simulink model "Grid_Connected_VSM"  (R2018a)
settings: Solver=ode45  StartTime=0.0  StopTime=0.6  RelTol=1e-3
InitFcn:
  | clear all;
  | Vdc = 1200;
  | fc = 10e3;
  | Rf = 0.07;
  | Lf = 5.2e-3;
  | Cf = 100e-6;
  | Lc = 1.5e-4;
  | Rc = 0.05;
  | Vref = sqrt(2/3)*400;
  | 
  | Kpv = 3;
  | Kiv = 400;
  | Kpc = 5;
  | Kic = 10;
  | 
  | 
  | J=0.05;
  | D=10;
  | %D = 1000;
  | wn=2*pi*50;
  | wf = 10*pi;
  | mq = 1e-5;
undefined symbols (not defined in the file): R2
libraries: powerlib x13, powerlib_meascontrol x5, simulink x4
settings Model: SimulationMode=accelerator  Creator=Deependra  LastModifiedBy=Deependra

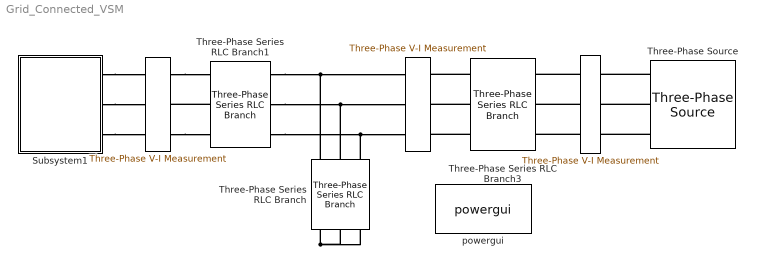
== system Grid_Connected_VSM ==
  " " : powerlib/Measurements/Three-Phase V-I Measurement  VoltageMeasurement=phase-to-ground  SetLabelV=on  LabelV=Viabc  Vpu=off  VpuLL=off  CurrentMeasurement=yes  SetLabelI=on  LabelI=ILabc  Ipu=off  Pbase=100e6  Vbase=500e3  OutputType=Complex  PhasorSimulation=off  PSBequivalent=0
  "   " : powerlib/Measurements/Three-Phase V-I Measurement  VoltageMeasurement=phase-to-ground  SetLabelV=on  LabelV=Voabc  Vpu=off  VpuLL=off  CurrentMeasurement=yes  SetLabelI=on  LabelI=Ioabc  Ipu=off  Pbase=Pnom  Vbase=380  OutputType=Complex  PhasorSimulation=off  PSBequivalent=0
  "     " : powerlib/Measurements/Three-Phase V-I Measurement  VoltageMeasurement=phase-to-ground  SetLabelV=on  LabelV=Vg  Vpu=off  VpuLL=off  CurrentMeasurement=no  SetLabelI=off  LabelI=Iabc_0  Ipu=off  Pbase=Pnom  Vbase=380  OutputType=Complex  PhasorSimulation=off  PSBequivalent=0
  Subsystem1 : Subsystem
  Three-Phase Series RLC Branch : powerlib/Elements/Three-Phase Series RLC Branch  LConnTagsString=A|B|C  RConnTagsString=A|B|C  BranchType=C  Resistance=R2  Inductance=1e-3  Capacitance=Cf  Measurements=Branch voltages
  Three-Phase Series RLC Branch1 : powerlib/Elements/Three-Phase Series RLC Branch  LConnTagsString=A|B|C  RConnTagsString=A|B|C  BranchType=RL  Resistance=Rf  Inductance=Lf  Capacitance=4.5e-3  Measurements=Branch voltages
  Three-Phase Series RLC Branch3 : powerlib/Elements/Three-Phase Series RLC Branch  LConnTagsString=A|B|C  RConnTagsString=A|B|C  BranchType=RL  Resistance=Rc  Inductance=Lc  Capacitance=1e-6  Measurements=None
  Three-Phase Source : powerlib/Electrical Sources/Three-Phase Source  InternalConnection=Yg  VoltagePhases=off  Voltage=400  PhaseAngle=0  Voltage_phases=[25e3 25e3 25e3]/sqrt(3)  PhaseAngles_phases=[0 -120 +120]  Frequency=50  NonIdealSource=off  SpecifyImpedance=off  Resistance=0.8929  Inductance=16.58e-3  ShortCircuitLevel=100e6  BaseVoltage=25e3  XRratio=7  BusType=swing  Pref=10e3  Qref=0  Prefabc=[10e3, 10e3, 10e3]  Qrefabc=[0, 0, 0]  Qmin=-inf  Qmax=inf
  powergui : powerlib/powergui  Priority=1  SimulationMode=Discrete  SampleTime=5e-6  frequency=60  Iterations=50  frequencyindice=0  Pbase=100e6  ErrMax=1e-4  UnitsV=kV  UnitsW=MW  buscounter=0  FunctionMessages=off  echomessages=off  EnableUseOfTLC=off  CurrentSourceSwitches=off  DisableSnubberDevices=off  DisableRonSwitches=off  DisableVfSwitches=off  DisplayEquations=off  SolverType=Tustin/Backward Euler (TBE)  Interpol=off  ExternalGateDelay=off  methode=off  Ts=100  x0status=zero  SPID=off  SwTol=0  HookPort=off  RestoreLinks=warning  ResistiveCurrentMeasurement=off  Frange=[0:2:500]  Ylog=off  Xlog=on  ShowGrid=off  save=off  variable=ZData  structure=Ni  ZoomFFT=off  StartTime=0.6  cycles=10  DisplayStyle=1  fundamental=50  FreqAxis=off  MaxFrequency=1000  frequencyindicesteady=1  RmsSteady=1  display=off
  connections:
  Three-Phase Series RLC Branch/LConn1 -- Three-Phase Series RLC Branch1/RConn1 -- "   "/LConn1
  Three-Phase Series RLC Branch/LConn3 -- Three-Phase Series RLC Branch1/RConn3 -- "   "/LConn3
  Three-Phase Series RLC Branch/RConn1 -- Three-Phase Series RLC Branch/RConn2 -- Three-Phase Series RLC Branch/RConn3
  Three-Phase Series RLC Branch/LConn2 -- Three-Phase Series RLC Branch1/RConn2 -- "   "/LConn2
  Three-Phase Series RLC Branch3/LConn3 -- "   "/RConn3
  Three-Phase Series RLC Branch3/LConn1 -- "   "/RConn1
  "     "/LConn2 -- Three-Phase Series RLC Branch3/RConn2
  "     "/LConn1 -- Three-Phase Series RLC Branch3/RConn1
  Three-Phase Series RLC Branch3/LConn2 -- "   "/RConn2
  "     "/LConn3 -- Three-Phase Series RLC Branch3/RConn3
  Subsystem1/RConn1 -- " "/LConn1
  Subsystem1/RConn2 -- " "/LConn2
  Subsystem1/RConn3 -- " "/LConn3
  Three-Phase Source/RConn2 -- "     "/RConn2
  Three-Phase Source/RConn1 -- "     "/RConn1
  Three-Phase Source/RConn3 -- "     "/RConn3
  " "/RConn1 -- Three-Phase Series RLC Branch1/LConn1
  Three-Phase Series RLC Branch1/LConn2 -- " "/RConn2
  " "/RConn3 -- Three-Phase Series RLC Branch1/LConn3

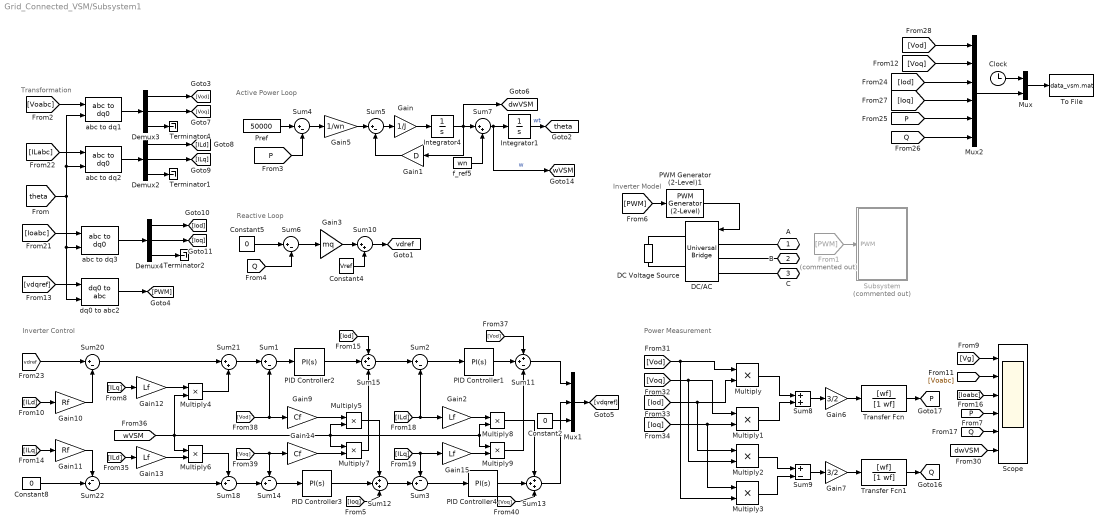
== system Grid_Connected_VSM/Subsystem1 ==
  note: Power Measurement
  note: Inverter Control
  note: Reactive Loop
  note: Transformation
  note: Active Power Loop
  note: Inverter Model
  Clock : Clock
  Constant2 : Constant  Value=0
  Constant4 : Constant  Value=Vref
  Constant5 : Constant  Value=0
  Constant8 : Constant  Value=0
  DC Voltage Source : powerlib/Electrical Sources/DC Voltage Source  Amplitude=Vdc  Measurements=None
  DC/AC : powerlib/Power Electronics/Universal Bridge  Arms=3  SnubberResistance=1e5  SnubberCapacitance=inf  Device=IGBT / Diodes  Ron=1e-3  Lon=0  ForwardVoltages="[  0  0  ]"  ForwardVoltage=0  GTOparameters=[ 10e-6 , 20e-6 ]  IGBTparameters=[ 1e-6 , 2e-6 ]  Measurements=None  Measurements_2=None  converterType=Rectifier
  Demux2 : Demux  Outputs=3
  Demux3 : Demux  Outputs=3
  Demux4 : Demux  Outputs=3
  From1 : From  Commented=on  GotoTag=PWM
  Gain : Gain  Gain=1/J
  Gain1 : Gain  Gain=D
  Gain10 : Gain  Gain=Rf
  Gain11 : Gain  Gain=Rf
  Gain{2,12..13,15} (4 alike) : Gain  Gain=Lf
  Gain14 : Gain  Gain=Cf
  Gain3 : Gain  Gain=mq
  Gain5 : Gain  Gain=1/wn
  Gain6 : Gain  Gain=3/2
  Gain7 : Gain  Gain=3/2
  Gain9 : Gain  Gain=Cf
  Integrator1 : Integrator
  Integrator4 : Integrator
  Multiply{,1..9} (10 alike) : Product
  Mux : Mux  Inputs=2
  Mux1 : Mux  Inputs=3
  Mux2 : Mux  Inputs=6
  PID Controller1 : simulink/Continuous/PID Controller  Controller=PI  TimeDomain=Continuous-time  SampleTime=-1  IntegratorMethod=Forward Euler  FilterMethod=Forward Euler  Form=Parallel  UseFilter=on  ControllerParametersSource=internal  P=Kpc  I=Kic  D=30  N=100  InitialConditionSource=internal  InitialConditionForIntegrator=0  InitialConditionForFilter=0  ExternalReset=none  LimitOutput=off  UpperSaturationLimit=inf  LowerSaturationLimit=-inf  LinearizeAsGain=on  AntiWindupMode=none  Kb=1  TrackingMode=off  Kt=1  PParamMin=[]  PParamMax=[]  IParamMin=[]  IParamMax=[]  DParamMin=[]  DParamMax=[]  NParamMin=[]  NParamMax=[]  KbParamMin=[]  KbParamMax=[]  KtParamMin=[]  KtParamMax=[]  POutMin=[]  POutMax=[]  IOutMin=[]  IOutMax=[]  DOutMin=[]  DOutMax=[]  NOutMin=[]  NOutMax=[]  KbOutMin=[]  KbOutMax=[]  KtOutMin=[]  KtOutMax=[]  IntegratorOutMin=[]  IntegratorOutMax=[]  FilterOutMin=[]  FilterOutMax=[]  SumOutMin=[]  SumOutMax=[]  SumI1OutMin=[]  SumI1OutMax=[]  SumI2OutMin=[]  SumI2OutMax=[]  SumI3OutMin=[]  SumI3OutMax=[]  SumDOutMin=[]  SumDOutMax=[]  SaturationOutMin=[]  SaturationOutMax=[]  IntegratorContinuousStateAttributes=''  IntegratorStateMustResolveToSignalObject=off  IntegratorRTWStateStorageClass=Auto  FilterContinuousStateAttributes=''  FilterStateMustResolveToSignalObject=off  FilterRTWStateStorageClass=Auto  DifferentiatorICPrevScaledInput=0  DifferentiatorOutMin=[]  DifferentiatorOutMax=[]  FilterDiffOutCoefMin=[]  FilterDiffOutCoefMax=[]  SumDenOutMin=[]  SumDenOutMax=[]  SumNumOutMin=[]  SumNumOutMax=[]  ReciprocalOutMin=[]  ReciprocalOutMax=[]  DivideOutMin=[]  DivideOutMax=[]  TunerSelectOption=Transfer Function Based (PID Tuner App)
  PID Controller2 : simulink/Continuous/PID Controller  Controller=PI  TimeDomain=Continuous-time  SampleTime=-1  IntegratorMethod=Forward Euler  FilterMethod=Forward Euler  Form=Parallel  UseFilter=on  ControllerParametersSource=internal  P=Kpv  I=Kiv  D=30  N=100  InitialConditionSource=internal  InitialConditionForIntegrator=0  InitialConditionForFilter=0  ExternalReset=none  LimitOutput=off  UpperSaturationLimit=inf  LowerSaturationLimit=-inf  LinearizeAsGain=on  AntiWindupMode=none  Kb=1  TrackingMode=off  Kt=1  PParamMin=[]  PParamMax=[]  IParamMin=[]  IParamMax=[]  DParamMin=[]  DParamMax=[]  NParamMin=[]  NParamMax=[]  KbParamMin=[]  KbParamMax=[]  KtParamMin=[]  KtParamMax=[]  POutMin=[]  POutMax=[]  IOutMin=[]  IOutMax=[]  DOutMin=[]  DOutMax=[]  NOutMin=[]  NOutMax=[]  KbOutMin=[]  KbOutMax=[]  KtOutMin=[]  KtOutMax=[]  IntegratorOutMin=[]  IntegratorOutMax=[]  FilterOutMin=[]  FilterOutMax=[]  SumOutMin=[]  SumOutMax=[]  SumI1OutMin=[]  SumI1OutMax=[]  SumI2OutMin=[]  SumI2OutMax=[]  SumI3OutMin=[]  SumI3OutMax=[]  SumDOutMin=[]  SumDOutMax=[]  SaturationOutMin=[]  SaturationOutMax=[]  IntegratorContinuousStateAttributes=''  IntegratorStateMustResolveToSignalObject=off  IntegratorRTWStateStorageClass=Auto  FilterContinuousStateAttributes=''  FilterStateMustResolveToSignalObject=off  FilterRTWStateStorageClass=Auto  DifferentiatorICPrevScaledInput=0  DifferentiatorOutMin=[]  DifferentiatorOutMax=[]  FilterDiffOutCoefMin=[]  FilterDiffOutCoefMax=[]  SumDenOutMin=[]  SumDenOutMax=[]  SumNumOutMin=[]  SumNumOutMax=[]  ReciprocalOutMin=[]  ReciprocalOutMax=[]  DivideOutMin=[]  DivideOutMax=[]  TunerSelectOption=Transfer Function Based (PID Tuner App)
  PID Controller3 : simulink/Continuous/PID Controller  Controller=PI  TimeDomain=Continuous-time  SampleTime=-1  IntegratorMethod=Forward Euler  FilterMethod=Forward Euler  Form=Parallel  UseFilter=on  ControllerParametersSource=internal  P=Kpv  I=Kiv  D=30  N=100  InitialConditionSource=internal  InitialConditionForIntegrator=0  InitialConditionForFilter=0  ExternalReset=none  LimitOutput=off  UpperSaturationLimit=inf  LowerSaturationLimit=-inf  LinearizeAsGain=on  AntiWindupMode=none  Kb=1  TrackingMode=off  Kt=1  PParamMin=[]  PParamMax=[]  IParamMin=[]  IParamMax=[]  DParamMin=[]  DParamMax=[]  NParamMin=[]  NParamMax=[]  KbParamMin=[]  KbParamMax=[]  KtParamMin=[]  KtParamMax=[]  POutMin=[]  POutMax=[]  IOutMin=[]  IOutMax=[]  DOutMin=[]  DOutMax=[]  NOutMin=[]  NOutMax=[]  KbOutMin=[]  KbOutMax=[]  KtOutMin=[]  KtOutMax=[]  IntegratorOutMin=[]  IntegratorOutMax=[]  FilterOutMin=[]  FilterOutMax=[]  SumOutMin=[]  SumOutMax=[]  SumI1OutMin=[]  SumI1OutMax=[]  SumI2OutMin=[]  SumI2OutMax=[]  SumI3OutMin=[]  SumI3OutMax=[]  SumDOutMin=[]  SumDOutMax=[]  SaturationOutMin=[]  SaturationOutMax=[]  IntegratorContinuousStateAttributes=''  IntegratorStateMustResolveToSignalObject=off  IntegratorRTWStateStorageClass=Auto  FilterContinuousStateAttributes=''  FilterStateMustResolveToSignalObject=off  FilterRTWStateStorageClass=Auto  DifferentiatorICPrevScaledInput=0  DifferentiatorOutMin=[]  DifferentiatorOutMax=[]  FilterDiffOutCoefMin=[]  FilterDiffOutCoefMax=[]  SumDenOutMin=[]  SumDenOutMax=[]  SumNumOutMin=[]  SumNumOutMax=[]  ReciprocalOutMin=[]  ReciprocalOutMax=[]  DivideOutMin=[]  DivideOutMax=[]  TunerSelectOption=Transfer Function Based (PID Tuner App)
  PID Controller4 : simulink/Continuous/PID Controller  Controller=PI  TimeDomain=Continuous-time  SampleTime=-1  IntegratorMethod=Forward Euler  FilterMethod=Forward Euler  Form=Parallel  UseFilter=on  ControllerParametersSource=internal  P=Kpc  I=Kic  D=30  N=100  InitialConditionSource=internal  InitialConditionForIntegrator=0  InitialConditionForFilter=0  ExternalReset=none  LimitOutput=off  UpperSaturationLimit=inf  LowerSaturationLimit=-inf  LinearizeAsGain=on  AntiWindupMode=none  Kb=1  TrackingMode=off  Kt=1  PParamMin=[]  PParamMax=[]  IParamMin=[]  IParamMax=[]  DParamMin=[]  DParamMax=[]  NParamMin=[]  NParamMax=[]  KbParamMin=[]  KbParamMax=[]  KtParamMin=[]  KtParamMax=[]  POutMin=[]  POutMax=[]  IOutMin=[]  IOutMax=[]  DOutMin=[]  DOutMax=[]  NOutMin=[]  NOutMax=[]  KbOutMin=[]  KbOutMax=[]  KtOutMin=[]  KtOutMax=[]  IntegratorOutMin=[]  IntegratorOutMax=[]  FilterOutMin=[]  FilterOutMax=[]  SumOutMin=[]  SumOutMax=[]  SumI1OutMin=[]  SumI1OutMax=[]  SumI2OutMin=[]  SumI2OutMax=[]  SumI3OutMin=[]  SumI3OutMax=[]  SumDOutMin=[]  SumDOutMax=[]  SaturationOutMin=[]  SaturationOutMax=[]  IntegratorContinuousStateAttributes=''  IntegratorStateMustResolveToSignalObject=off  IntegratorRTWStateStorageClass=Auto  FilterContinuousStateAttributes=''  FilterStateMustResolveToSignalObject=off  FilterRTWStateStorageClass=Auto  DifferentiatorICPrevScaledInput=0  DifferentiatorOutMin=[]  DifferentiatorOutMax=[]  FilterDiffOutCoefMin=[]  FilterDiffOutCoefMax=[]  SumDenOutMin=[]  SumDenOutMax=[]  SumNumOutMin=[]  SumNumOutMax=[]  ReciprocalOutMin=[]  ReciprocalOutMax=[]  DivideOutMin=[]  DivideOutMax=[]  TunerSelectOption=Transfer Function Based (PID Tuner App)
  PWM Generator (2-Level)1 : powerlib_meascontrol/Pulse & Signal Generators/PWM Generator (2-Level)  ModulatorType=Three-phase bridge (6 pulses)  ModulatorMode=Unsynchronized  Fc=fc  Pc=0  nF=27  MinMax="[ -1  1 ]"  SamplingTechnique=Natural  ModulatingSignals=off  m=0.8  Freq=60  Phase=0  Ts=0  ShowCarrierOutport=off
      settings: SourceProductName=Simscape Power Systems
  Pref : Constant  Value=50000
  Scope : Scope  NumInputPorts=6
  Subsystem : Subsystem  Commented=on
  Sum{1..2,4..6,20} (6 alike) : Sum  Inputs=|+-
  Sum10 : Sum  Inputs=|++
  Sum11 : Sum  Inputs=++-
  Sum12 : Sum  Inputs=+++
  Sum13 : Sum  Inputs=+++
  Sum{3,14,18,22} (4 alike) : Sum  Inputs=-+|
  Sum15 : Sum  Inputs=++-
  Sum21 : Sum  Inputs=|++
  Sum7 : Sum  Inputs=|++
  Sum8 : Sum
  Sum9 : Sum  Inputs=+-
  Terminator1 : Terminator
  Terminator2 : Terminator
  Terminator4 : Terminator
  To File : ToFile  Filename=data_vsm.mat  SampleTime=0.00001
  Transfer Fcn : TransferFcn  Numerator=[wf]  Denominator=[1 wf]
  Transfer Fcn1 : TransferFcn  Numerator=[wf]  Denominator=[1 wf]
  abc to dq1 : powerlib_meascontrol/Transformations/abc to dq0  Alignment=90 degrees behind phase A axis
  abc to dq2 : powerlib_meascontrol/Transformations/abc to dq0  Alignment=90 degrees behind phase A axis
  abc to dq3 : powerlib_meascontrol/Transformations/abc to dq0  Alignment=90 degrees behind phase A axis
  dq0 to abc2 : powerlib_meascontrol/Transformations/dq0 to abc  Alignment=90 degrees behind phase A axis
  f_ref5 : Constant  Value=wn
  A : PMIOPort  Side=Right
  B : PMIOPort  Port=2  Side=Right
  C : PMIOPort  Port=3  Side=Right
  tag scope: P=global, Q=global, dwVSM=global, theta=global, vdref=global, wVSM=global
  wires:
  From1/1 -> Subsystem/1(PWM)
  Pref/1 -> Sum4/1
  Sum7/1 -> [wVSM], Integrator1/1  "w"
  Sum4/1 -> Gain5/1
  Gain5/1 -> Sum5/1
  Sum5/1 -> Gain/1
  Integrator4/1 -> [dwVSM], Sum7/1, Gain1/1
  f_ref5/1 -> Sum7/2
  Integrator1/1 -> [theta]  "wt"
  [P] -> Sum4/2
  Gain1/1 -> Sum5/2
  Gain/1 -> Integrator4/1
  Demux3/1 -> [Vod]
  Demux4/2 -> [Ioq]
  Demux4/1 -> [Iod]
  abc to dq2/1 -> Demux2/1
  [ILabc] -> abc to dq2/1
  Demux2/1 -> [ILd]
  abc to dq3/1 -> Demux4/1
  Demux4/3 -> Terminator2/1
  Demux3/3 -> Terminator4/1
  Demux2/3 -> Terminator1/1
  Demux2/2 -> [ILq]
  [Ioabc] -> abc to dq3/1
  [Iod] -> Multiply2/1, Multiply/2
  Multiply/1 -> Sum8/1
  Multiply1/1 -> Sum8/2
  Transfer Fcn/1 -> [P]
  Multiply2/1 -> Sum9/1
  Transfer Fcn1/1 -> [Q]
  Sum9/1 -> Gain7/1
  Gain6/1 -> Transfer Fcn/1
  Multiply3/1 -> Sum9/2
  [Voq] -> Multiply2/2, Multiply1/1
  [Vod] -> Multiply3/2, Multiply/1
  Gain7/1 -> Transfer Fcn1/1
  Sum8/1 -> Gain6/1
  [Ioq] -> Multiply3/1, Multiply1/2
  [Voabc] -> Scope/2
  Sum10/1 -> [vdref]
  [Q] -> Scope/5
  [Vg] -> Scope/1
  [Ioabc] -> Scope/3
  [P] -> Scope/4
  [dwVSM] -> Scope/6
  Gain3/1 -> Sum10/1
  Sum6/1 -> Gain3/1
  Constant4/1 -> Sum10/2
  [Q] -> Sum6/2
  Constant5/1 -> Sum6/1
  PWM Generator (2-Level)1/1 -> DC/AC/1
  [PWM] -> PWM Generator (2-Level)1/1
  [ILq] -> Gain12/1
  Gain10/1 -> Sum20/2
  [vdref] -> Sum20/1
  Multiply6/1 -> Sum18/1
  [ILd] -> Gain10/1
  Gain13/1 -> Multiply6/2
  Sum22/1 -> Sum18/2
  [ILd] -> Gain13/1
  Gain12/1 -> Multiply4/1
  Multiply4/1 -> Sum21/2
  Constant8/1 -> Sum22/2
  Sum20/1 -> Sum21/1
  [ILq] -> Gain11/1
  Gain11/1 -> Sum22/1
  Sum21/1 -> Sum1/1
  [ILq] -> Gain15/1, Sum3/1
  Gain2/1 -> Multiply8/1
  [Vod] -> Sum11/1
  Sum12/1 -> Sum3/2
  Sum2/1 -> PID Controller1/1
  [ILd] -> Gain2/1, Sum2/2
  PID Controller2/1 -> Sum15/2
  Sum14/1 -> PID Controller3/1
  Sum3/1 -> PID Controller4/1
  [Ioq] -> Sum12/3
  [Voq] -> Sum13/3
  [Iod] -> Sum15/1
  Gain9/1 -> Multiply5/1
  Multiply7/1 -> Sum15/3
  Multiply5/1 -> Sum12/1
  PID Controller4/1 -> Sum13/2
  [Voq] -> Gain14/1, Sum14/1
  Multiply9/1 -> Sum11/3
  [wVSM] -> Multiply4/2, Multiply7/1, Multiply9/1, Multiply8/2, Multiply5/2, Multiply6/1
  Sum11/1 -> Mux1/1
  Gain14/1 -> Multiply7/2
  PID Controller3/1 -> Sum12/2
  [Vod] -> Sum1/2, Gain9/1
  Constant2/1 -> Mux1/3
  Sum13/1 -> Mux1/2
  Sum18/1 -> Sum14/2
  PID Controller1/1 -> Sum11/2
  Sum1/1 -> PID Controller2/1
  Sum15/1 -> Sum2/1
  Multiply8/1 -> Sum13/1
  Gain15/1 -> Multiply9/2
  Mux1/1 -> [vdqref]
  [vdqref] -> dq0 to abc2/1
  [theta] -> abc to dq1/2, abc to dq2/2, abc to dq3/2, dq0 to abc2/2
  [P] -> Mux2/5
  [Voq] -> Mux2/2
  Clock/1 -> Mux/1
  [Vod] -> Mux2/1
  [Ioq] -> Mux2/4
  Mux2/1 -> Mux/2
  [Iod] -> Mux2/3
  Mux/1 -> To File/1
  [Q] -> Mux2/6
  [Voabc] -> abc to dq1/1
  abc to dq1/1 -> Demux3/1
  Demux3/2 -> [Voq]
  dq0 to abc2/1 -> [PWM]
  connections:
  DC/AC/RConn2 -- DC Voltage Source/LConn1
  DC/AC/RConn1 -- DC Voltage Source/RConn1
  DC/AC/LConn1 -- A/RConn1
  DC/AC/LConn2 -- B/RConn1
  DC/AC/LConn3 -- C/RConn1

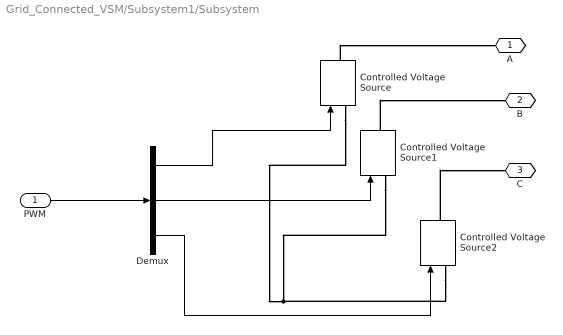
== system Grid_Connected_VSM/Subsystem1/Subsystem ==
  PWM : Inport
  Controlled Voltage Source : powerlib/Electrical Sources/Controlled Voltage Source  Initialize=off  Source_Type=AC  Amplitude=0  Phase=0  Frequency=0  Measurements=None
  Controlled Voltage Source1 : powerlib/Electrical Sources/Controlled Voltage Source  Initialize=off  Source_Type=AC  Amplitude=0  Phase=0  Frequency=0  Measurements=None
  Controlled Voltage Source2 : powerlib/Electrical Sources/Controlled Voltage Source  Initialize=off  Source_Type=AC  Amplitude=0  Phase=0  Frequency=0  Measurements=None
  Demux : Demux  Outputs=3
  A : PMIOPort  Side=Right
  B : PMIOPort  Port=2  Side=Right
  C : PMIOPort  Port=3  Side=Right
  wires:
  PWM/1 -> Demux/1
  Demux/1 -> Controlled Voltage Source/1
  Demux/2 -> Controlled Voltage Source1/1
  Demux/3 -> Controlled Voltage Source2/1
  connections:
  Controlled Voltage Source2/RConn1 -- C/RConn1
  Controlled Voltage Source/LConn1 -- Controlled Voltage Source1/LConn1 -- Controlled Voltage Source2/LConn1
  Controlled Voltage Source/RConn1 -- A/RConn1
  Controlled Voltage Source1/RConn1 -- B/RConn1
